simulink model "DiagramaSistemaCombinado"  (R2017b)
settings: Solver=VariableStepAuto  StartTime=0.0  StopTime=10.0  RelTol=1e-3
values from neighbouring files (symbols this model uses):
  B = 0.002953    [Graficas.m]
  Bl = 0.01    [Graficas.m]
  J = 0.0221    [Graficas.m]
  Jl = 0.125    [Graficas.m]
  Kb = 1.25    [Graficas.m]
  Kt = 0.516    [Graficas.m]
  L = 0.0281    [Graficas.m]
  n = N1/N2    (= 0.5)    [Graficas.m]
  R = 2.581    [Graficas.m]
  ST = 1    [Graficas.m]
  VF = 240    [Graficas.m]
  VI = 140    [Graficas.m]
settings Model: Creator=usuario  LastModifiedBy=Wilmer
settings SFSimCC: SimUseLocalCustomCode=on
settings RTWCC: RTWUseLocalCustomCode=on
settings CodeAppCC: StateflowObjectComments=on

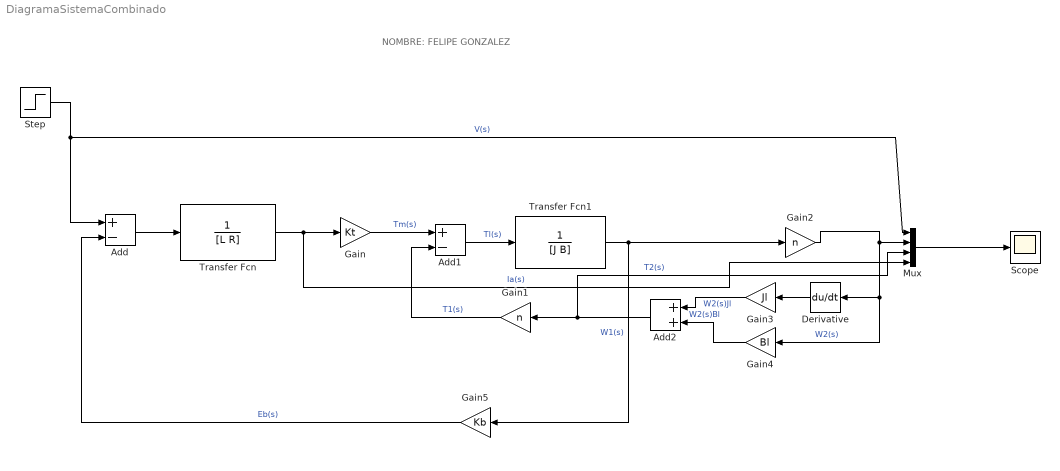
== system DiagramaSistemaCombinado ==
  note: NOMBRE: FELIPE GONZALEZ
  Add : Sum  Inputs=+-
  Add1 : Sum  Inputs=+-
  Add2 : Sum
  Derivative : Derivative
  Gain : Gain  Gain=Kt
  Gain1 : Gain  Gain=n
  Gain2 : Gain  Gain=n
  Gain3 : Gain  Gain=Jl
  Gain4 : Gain  Gain=Bl
  Gain5 : Gain  Gain=Kb
  Mux : Mux
  Scope : Scope
  Step : Step  Time=ST  Before=VI  After=VF  SampleTime=0
  Transfer Fcn : TransferFcn  Denominator=[L R]
  Transfer Fcn1 : TransferFcn  Denominator=[J B]
  wires:
  Add/1 -> Transfer Fcn/1
  Transfer Fcn/1 -> Mux/4, Gain/1  "Ia(s)"
  Gain/1 -> Add1/1  "Tm(s)"
  Add1/1 -> Transfer Fcn1/1  "Tl(s)"
  Gain1/1 -> Add1/2  "T1(s)"
  Transfer Fcn1/1 -> Gain5/1, Gain2/1  "W1(s)"
  Gain2/1 -> Gain4/1, Derivative/1, Mux/2  "W2(s)"
  Add2/1 -> Mux/3, Gain1/1  "T2(s)"
  Gain4/1 -> Add2/2  "W2(s)Bl"
  Gain3/1 -> Add2/1  "W2(s)Jl"
  Derivative/1 -> Gain3/1
  Gain5/1 -> Add/2  "Eb(s)"
  Step/1 -> Add/1, Mux/1  "V(s)"
  Mux/1 -> Scope/1
